simulink model "GuytonModel1986All_R2015a"  (R2015a)
settings: Solver=ode15s  StartTime=0  StopTime=383040  FixedStep=0.03  MaxStep=360  RelTol=1e-3
libraries: simulink x3
(part 4 of 5)

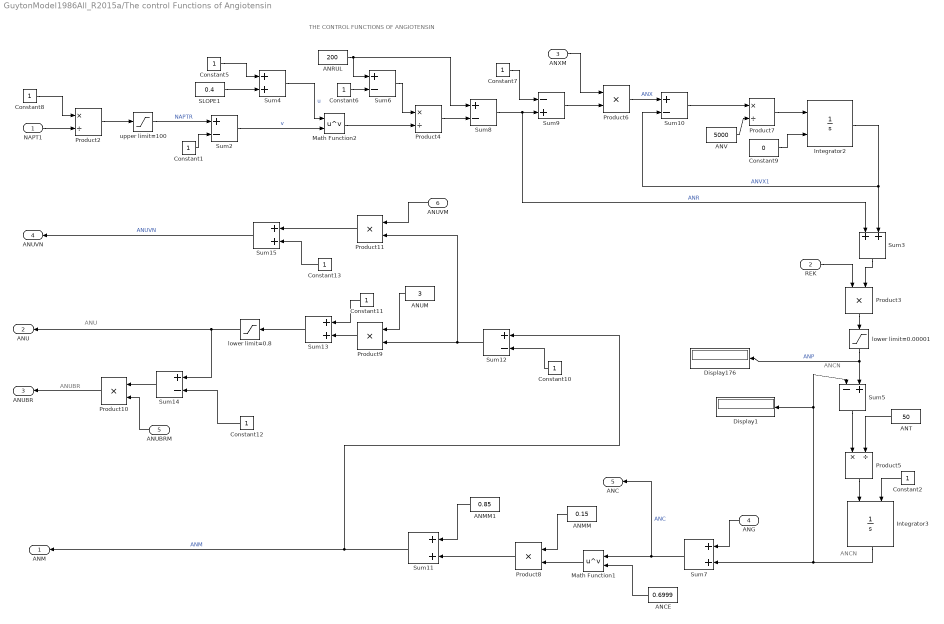
== system GuytonModel1986All_R2015a/The control Functions of Angiotensin ==
  note: THE CONTROL FUNCTIONS OF ANGIOTENSIN
  note: ANCN
  note: ANCN
  note: ANUBR
  note: ANU
  NAPT1 : Inport
  REK : Inport  Port=2
  ANXM : Inport  Port=3
  ANG : Inport  Port=4
  ANUBRM : Inport  Port=5
  ANUVM : Inport  Port=6
  ANCE : Constant  Value=0.6999
  ANMM : Constant  Value=0.15
  ANMM1 : Constant  Value=0.85
  ANRUL : Constant  Value=200
  ANT : Constant  Value=50
  ANUM : Constant  Value=3
  ANV : Constant  Value=5000
  Constant{1..2,5..8,10..13} (10 alike) : Constant
  Constant9 : Constant  Value=0
  Display1 : Display
  Display176 : Display
  Integrator2 : Integrator  InitialConditionSource=external
  Integrator3 : Integrator  InitialConditionSource=external
  Math Function1 : Math  Operator=pow  SaturateOnIntegerOverflow=on
  Math Function2 : Math  Operator=pow  SaturateOnIntegerOverflow=on
  Product{3,6,8..11} (6 alike) : Product  SaturateOnIntegerOverflow=on  RndMeth=Zero  InputSameDT=on  OutDataTypeStr=Inherit: Same as first input
  Product{2,4..5,7} (4 alike) : Product  Inputs=*/  SaturateOnIntegerOverflow=on  RndMeth=Zero  InputSameDT=on  OutDataTypeStr=Inherit: Same as first input
  SLOPE1 : Constant  Value=0.4
  Sum{2,6,8,10,12,14} (6 alike) : Sum  Inputs=+-  SaturateOnIntegerOverflow=on  InputSameDT=on  OutDataTypeStr=Inherit: Same as first input
  Sum11 : Sum  SaturateOnIntegerOverflow=on  InputSameDT=on  OutDataTypeStr=Inherit: Same as first input
  Sum13 : Sum  Inputs=2  SaturateOnIntegerOverflow=on  InputSameDT=on  OutDataTypeStr=Inherit: Same as first input
  Sum15 : Sum  SaturateOnIntegerOverflow=on  InputSameDT=on  OutDataTypeStr=Inherit: Same as first input
  Sum3 : Sum  Inputs=2  SaturateOnIntegerOverflow=on  InputSameDT=on  OutDataTypeStr=Inherit: Same as first input
  Sum4 : Sum  Inputs=2  SaturateOnIntegerOverflow=on  InputSameDT=on  OutDataTypeStr=Inherit: Same as first input
  Sum5 : Sum  Inputs=-+  SaturateOnIntegerOverflow=on  InputSameDT=on  OutDataTypeStr=Inherit: Same as first input
  Sum7 : Sum  SaturateOnIntegerOverflow=on  InputSameDT=on  OutDataTypeStr=Inherit: Same as first input
  Sum9 : Sum  Inputs=-+  SaturateOnIntegerOverflow=on  InputSameDT=on  OutDataTypeStr=Inherit: Same as first input
  lower limit=0.00001 : Saturate  UpperLimit=inf  LowerLimit=0.00001  LinearizeAsGain=off
  lower limit=0.8 : Saturate  UpperLimit=inf  LowerLimit=0.8  LinearizeAsGain=off
  "upper limit=100 " : Saturate  UpperLimit=100  LowerLimit=-inf  LinearizeAsGain=off
  ANM : Outport
  ANU : Outport  Port=2
  ANUBR : Outport  Port=3
  ANUVN : Outport  Port=4
  ANC : Outport  Port=5
  wires:
  NAPT1/1 -> Product2/2
  Constant8/1 -> Product2/1
  Product2/1 -> "upper limit=100 "/1
  "upper limit=100 "/1 -> Sum2/1  "NAPTR"
  Constant1/1 -> Sum2/2
  SLOPE1/1 -> Sum4/2
  Constant5/1 -> Sum4/1
  Sum4/1 -> Math Function2/1  "u"
  Sum2/1 -> Math Function2/2  "v"
  Constant6/1 -> Sum6/2
  ANRUL/1 -> Sum6/1, Sum8/1
  Math Function2/1 -> Product4/2
  Sum6/1 -> Product4/1
  Product4/1 -> Sum8/2
  Sum8/1 -> Sum9/2, Sum3/1  "ANR"
  Constant7/1 -> Sum9/1
  Sum9/1 -> Product6/2
  ANXM/1 -> Product6/1
  Product6/1 -> Sum10/1  "ANX"
  Sum10/1 -> Product7/1
  ANV/1 -> Product7/2
  Product7/1 -> Integrator2/1
  Constant9/1 -> Integrator2/2
  Integrator2/1 -> Sum10/2, Sum3/2  "ANVX1"
  Sum3/1 -> Product3/2
  REK/1 -> Product3/1
  Product3/1 -> lower limit=0.00001/1
  lower limit=0.00001/1 -> Sum5/2, Display176/1  "ANP"
  Sum5/1 -> Product5/1
  ANT/1 -> Product5/2
  Constant2/1 -> Integrator3/2
  Product5/1 -> Integrator3/1
  Integrator3/1 -> Sum7/2, Sum5/1, Display1/1
  ANG/1 -> Sum7/1
  Sum7/1 -> Math Function1/1, ANC/1  "ANC"
  ANCE/1 -> Math Function1/2
  Math Function1/1 -> Product8/2
  ANMM/1 -> Product8/1
  Product8/1 -> Sum11/2
  ANMM1/1 -> Sum11/1
  Sum11/1 -> Sum12/1, ANM/1  "ANM"
  Constant10/1 -> Sum12/2
  Sum12/1 -> Product9/2, Product11/2
  ANUM/1 -> Product9/1
  Product9/1 -> Sum13/2
  Constant11/1 -> Sum13/1
  Sum13/1 -> lower limit=0.8/1
  lower limit=0.8/1 -> Sum14/1, ANU/1
  Constant12/1 -> Sum14/2
  Sum14/1 -> Product10/1
  ANUBRM/1 -> Product10/2
  Product10/1 -> ANUBR/1
  ANUVM/1 -> Product11/1
  Constant13/1 -> Sum15/2
  Product11/1 -> Sum15/1
  Sum15/1 -> ANUVN/1  "ANUVN"

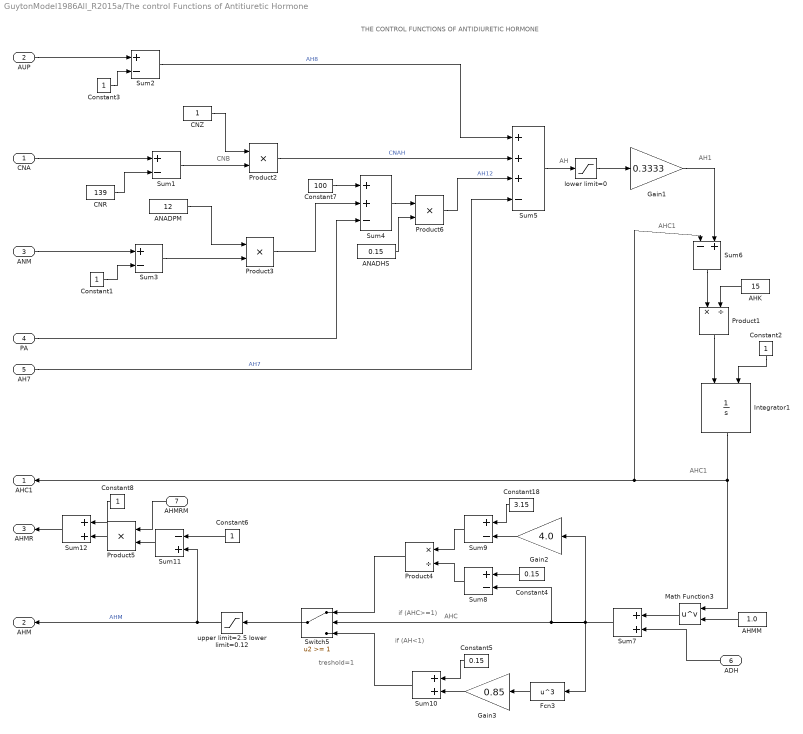
== system GuytonModel1986All_R2015a/The control Functions of Antitiuretic Hormone ==
  note: THE CONTROL FUNCTIONS OF ANTIDIURETIC HORMONE
  note: CNB
  note: AH
  note: AHC1
  note: AHC1
  note: treshold=1
  note: AHC
  note: if (AHC>=1)
  note: if (AH<1)
  note: AH1
  CNA : Inport
  AUP : Inport  Port=2
  ANM : Inport  Port=3
  PA : Inport  Port=4
  AH7 : Inport  Port=5
  ADH : Inport  Port=6
  AHMRM : Inport  Port=7
  AHK : Constant  Value=15
  AHMM : Constant  Value=1.0
  ANADHS : Constant  Value=0.15
  ANADPM : Constant  Value=12
  CNR : Constant  Value=139
  CNZ : Constant
  Constant{1..3,6,8} (5 alike) : Constant
  Constant18 : Constant  Value=3.15
  Constant4 : Constant  Value=0.15
  Constant5 : Constant  Value=0.15
  Constant7 : Constant  Value=100
  Fcn3 : Fcn  Expr=u^3
  Gain1 : Gain  Gain=0.3333  SaturateOnIntegerOverflow=on  OutDataTypeStr=Inherit: Same as input  ParamDataTypeStr=Inherit: Same as input
  Gain2 : Gain  Gain=4.0  SaturateOnIntegerOverflow=on  OutDataTypeStr=Inherit: Same as input  ParamDataTypeStr=Inherit: Same as input
  Gain3 : Gain  Gain=0.85  SaturateOnIntegerOverflow=on  OutDataTypeStr=Inherit: Same as input  ParamDataTypeStr=Inherit: Same as input
  Integrator1 : Integrator  InitialConditionSource=external
  Math Function3 : Math  Operator=pow  SaturateOnIntegerOverflow=on
  Product1 : Product  Inputs=*/  SaturateOnIntegerOverflow=on  RndMeth=Zero  InputSameDT=on  OutDataTypeStr=Inherit: Same as first input
  Product{2..3,5..6} (4 alike) : Product  SaturateOnIntegerOverflow=on  RndMeth=Zero  InputSameDT=on  OutDataTypeStr=Inherit: Same as first input
  Product4 : Product  Inputs=*/  SaturateOnIntegerOverflow=on  RndMeth=Zero  InputSameDT=on  OutDataTypeStr=Inherit: Same as first input
  Sum{1..3,8..9} (5 alike) : Sum  Inputs=+-  SaturateOnIntegerOverflow=on  InputSameDT=on  OutDataTypeStr=Inherit: Same as first input
  Sum10 : Sum  Inputs=2  SaturateOnIntegerOverflow=on  InputSameDT=on  OutDataTypeStr=Inherit: Same as first input
  Sum11 : Sum  Inputs=-+  SaturateOnIntegerOverflow=on  InputSameDT=on  OutDataTypeStr=Inherit: Same as first input
  Sum12 : Sum  Inputs=2  SaturateOnIntegerOverflow=on  InputSameDT=on  OutDataTypeStr=Inherit: Same as first input
  Sum4 : Sum  Inputs=++-  SaturateOnIntegerOverflow=on  InputSameDT=on  OutDataTypeStr=Inherit: Same as first input
  Sum5 : Sum  Inputs=+++-  SaturateOnIntegerOverflow=on  InputSameDT=on  OutDataTypeStr=Inherit: Same as first input
  Sum6 : Sum  Inputs=-+  SaturateOnIntegerOverflow=on  InputSameDT=on  OutDataTypeStr=Inherit: Same as first input
  Sum7 : Sum  Inputs=2  SaturateOnIntegerOverflow=on  InputSameDT=on  OutDataTypeStr=Inherit: Same as first input
  Switch5 : Switch  Threshold=1  SaturateOnIntegerOverflow=on  InputSameDT=on
  "lower limit=0 " : Saturate  UpperLimit=inf  LowerLimit=0  LinearizeAsGain=off
  "upper limit=2.5 lower limit=0.12 " : Saturate  UpperLimit=inf  LowerLimit=0  LinearizeAsGain=off
  AHC1 : Outport
  AHM : Outport  Port=2
  AHMR : Outport  Port=3
  wires:
  CNR/1 -> Sum1/2
  CNA/1 -> Sum1/1
  Sum1/1 -> Product2/2
  CNZ/1 -> Product2/1
  Constant3/1 -> Sum2/2
  AUP/1 -> Sum2/1
  Constant1/1 -> Sum3/2
  ANM/1 -> Sum3/1
  Sum3/1 -> Product3/2
  ANADPM/1 -> Product3/1
  Product3/1 -> Sum4/2
  PA/1 -> Sum4/3
  Sum2/1 -> Sum5/1  "AH8"
  Constant7/1 -> Sum4/1
  Product2/1 -> Sum5/2  "CNAH"
  AH7/1 -> Sum5/4  "AH7"
  Sum5/1 -> "lower limit=0 "/1
  "lower limit=0 "/1 -> Gain1/1
  Constant2/1 -> Integrator1/2
  AHK/1 -> Product1/2
  Sum6/1 -> Product1/1
  Product1/1 -> Integrator1/1
  Integrator1/1 -> Sum6/1, AHC1/1, Math Function3/1
  Gain1/1 -> Sum6/2
  AHMM/1 -> Math Function3/2
  Math Function3/1 -> Sum7/1
  ADH/1 -> Sum7/2
  Sum7/1 -> Switch5/2, Sum8/2, Gain2/1, Fcn3/1
  Constant4/1 -> Sum8/1
  Gain2/1 -> Sum9/2
  Constant18/1 -> Sum9/1
  Sum9/1 -> Product4/1
  Sum8/1 -> Product4/2
  Product4/1 -> Switch5/1
  Fcn3/1 -> Gain3/1
  Gain3/1 -> Sum10/2
  Constant5/1 -> Sum10/1
  Sum10/1 -> Switch5/3
  Switch5/1 -> "upper limit=2.5 lower limit=0.12 "/1
  "upper limit=2.5 lower limit=0.12 "/1 -> AHM/1, Sum11/2  "AHM"
  Constant6/1 -> Sum11/1
  Sum11/1 -> Product5/2
  AHMRM/1 -> Product5/1
  Product5/1 -> Sum12/2
  Constant8/1 -> Sum12/1
  Sum12/1 -> AHMR/1
  Sum4/1 -> Product6/1
  Product6/1 -> Sum5/3  "AH12"
  ANADHS/1 -> Product6/2

== system GuytonModel1986All_R2015a/The volume receptor feedback mechanism ==
  note: PRA
  note: AHZ1
  note: ATRVFB
  note: ATRRFB
  note: AH7
  note: Dumping
  note: The volume receptor feedback mechanism
  PRA : Inport
  ATRVFBM : Inport  Port=2
  ATRRFBM : Inport  Port=3
  "AH10 " : Constant  Value=0.333
  AH11 : Constant  Value=1000
  AH9 : Constant
  AHY : Integrator  InitialConditionSource=external
  AHY0 : Constant  Value=0
  AHY1 : Constant  Value=0.1
  AHZ1=(Abs(PRA))^AH10 : Math  Operator=pow  SaturateOnIntegerOverflow=on
  "ATRVFB " : Integrator  InitialConditionSource=external
  ATRVFB0 : Constant  Value=0
  ATRVFB1 : Constant  Value=0.1
  Abs : Abs  SaturateOnIntegerOverflow=on
  Constant12 : Constant
  Gain1 : Gain  Gain=-1  SaturateOnIntegerOverflow=on  OutDataTypeStr=Inherit: Same as input  ParamDataTypeStr=Inherit: Same as input
  Product{1,4..6} (4 alike) : Product  SaturateOnIntegerOverflow=on  RndMeth=Zero  InputSameDT=on  OutDataTypeStr=Inherit: Same as first input
  Product9 : Product  Inputs=*/  SaturateOnIntegerOverflow=on  RndMeth=Zero  InputSameDT=on  OutDataTypeStr=Inherit: Same as first input
  Sum1 : Sum  Inputs=+-  SaturateOnIntegerOverflow=on  InputSameDT=on  OutDataTypeStr=Inherit: Same as first input
  Sum6 : Sum  Inputs=+-  SaturateOnIntegerOverflow=on  InputSameDT=on  OutDataTypeStr=Inherit: Same as first input
  Sum7 : Sum  SaturateOnIntegerOverflow=on  InputSameDT=on  OutDataTypeStr=Inherit: Same as first input
  Sum9 : Sum  Inputs=+-  SaturateOnIntegerOverflow=on  InputSameDT=on  OutDataTypeStr=Inherit: Same as first input
  if (ATRRFB)>=0.!) ATRRFB=ATRRFB else ATRRFB= 0.1 : Switch  Threshold=0.1  SaturateOnIntegerOverflow=on  InputSameDT=on
  "if (PRA>=0) AHZ2=AHZ1 else AHZ2= -AHZ1  " : Switch  SaturateOnIntegerOverflow=on  InputSameDT=on
  AH7 : Outport
  ATRVFB : Outport  Port=2
  ATRRFB : Outport  Port=3
  wires:
  Product1/1 -> "ATRVFB "/1
  ATRVFB1/1 -> Product1/2
  "ATRVFB "/1 -> Sum1/2, ATRVFB/1
  Sum1/1 -> Product1/1
  ATRVFB0/1 -> "ATRVFB "/2
  "AH10 "/1 -> AHZ1=(Abs(PRA))^AH10/2
  Abs/1 -> AHZ1=(Abs(PRA))^AH10/1
  AH11/1 -> Product9/2
  AHY0/1 -> AHY/2
  ATRRFBM/1 -> Product5/1
  PRA/1 -> "if (PRA>=0) AHZ2=AHZ1 else AHZ2= -AHZ1  "/2, Abs/1  "PRA"
  Product6/1 -> Sum1/1
  ATRVFBM/1 -> Product6/1
  Constant12/1 -> Sum7/1
  Product5/1 -> Sum7/2
  AH9/1 -> Product4/1
  Gain1/1 -> "if (PRA>=0) AHZ2=AHZ1 else AHZ2= -AHZ1  "/3  "-AHZ1"
  AHZ1=(Abs(PRA))^AH10/1 -> "if (PRA>=0) AHZ2=AHZ1 else AHZ2= -AHZ1  "/1, Gain1/1  "AHZ1"
  Sum6/1 -> AH7/1, Product6/2, Product5/2
  Product4/1 -> Sum9/1, Sum6/1  "AHZ"
  Sum9/1 -> Product9/1
  "if (PRA>=0) AHZ2=AHZ1 else AHZ2= -AHZ1  "/1 -> Product4/2
  AHY/1 -> Sum9/2, Sum6/2
  Product9/1 -> AHY/1
  AHY1/1 -> if (ATRRFB)>=0.!) ATRRFB=ATRRFB else ATRRFB= 0.1/3
  Sum7/1 -> if (ATRRFB)>=0.!) ATRRFB=ATRRFB else ATRRFB= 0.1/2, if (ATRRFB)>=0.!) ATRRFB=ATRRFB else ATRRFB= 0.1/1
  if (ATRRFB)>=0.!) ATRRFB=ATRRFB else ATRRFB= 0.1/1 -> ATRRFB/1

== system GuytonModel1986All_R2015a/Thirst, Drinking and Salt Appetite ==
  note: If TVD <0 then TVD=DR
  note: If STHENABLED <0 then STH=1
  note: TVZ
  note: ANMTH
  note: THIRST, DRINKING AND SALT APPETITE
  POT : Inport
  AHC1 : Inport  Port=2
  ANM : Inport  Port=3
  DR : Inport  Port=4
  STHENABLED : Inport  Port=5
  TVDENABLED : Inport  Port=6
  AHTHM : Constant  Value=2
  ANMTM : Constant  Value=1.5
  Constant{1..3,8} (4 alike) : Constant
  Constant4 : Constant  Value=0.001
  Display4 : Display
  Gain1 : Gain  Gain=0.001  SaturateOnIntegerOverflow=on  OutDataTypeStr=Inherit: Same as input  ParamDataTypeStr=Inherit: Same as input
  Gain2 : Gain  Gain=0.001  SaturateOnIntegerOverflow=on  OutDataTypeStr=Inherit: Same as input  ParamDataTypeStr=Inherit: Same as input
  Integrator1 : Integrator  InitialConditionSource=external
  Product{1..5} (5 alike) : Product  SaturateOnIntegerOverflow=on  RndMeth=Zero  InputSameDT=on  OutDataTypeStr=Inherit: Same as first input
  Sum1 : Sum  Inputs=+-  SaturateOnIntegerOverflow=on  InputSameDT=on  OutDataTypeStr=Inherit: Same as first input
  Sum2 : Sum  Inputs=+-  SaturateOnIntegerOverflow=on  InputSameDT=on  OutDataTypeStr=Inherit: Same as first input
  Sum3 : Sum  SaturateOnIntegerOverflow=on  InputSameDT=on  OutDataTypeStr=Inherit: Same as first input
  Sum5 : Sum  SaturateOnIntegerOverflow=on  InputSameDT=on  OutDataTypeStr=Inherit: Same as first input
  Sum6 : Sum  Inputs=+-  SaturateOnIntegerOverflow=on  InputSameDT=on  OutDataTypeStr=Inherit: Same as first input
  Sum7 : Sum  Inputs=-++  SaturateOnIntegerOverflow=on  InputSameDT=on  OutDataTypeStr=Inherit: Same as first input
  TRESHOLD=0 : Switch  Criteria=u2 > Threshold
  "TRESHOLD=0 " : Switch  Criteria=u2 > Threshold
  TVDDL : Constant  Value=30
  Z10 : Constant  Value=8.25
  Z11 : Constant  Value=4
  lower limit=0 : Saturate  UpperLimit=inf  LowerLimit=0  LinearizeAsGain=off
  "lower limit=0 " : Saturate  UpperLimit=inf  LowerLimit=0  LinearizeAsGain=off
  "upper limit=8 lower limit=1 " : Saturate  UpperLimit=8  LowerLimit=1  LinearizeAsGain=off
  STH : Outport
  TVD : Outport  Port=2
  wires:
  TVDENABLED/1 -> "TRESHOLD=0 "/2
  "TRESHOLD=0 "/1 -> TVD/1
  STHENABLED/1 -> TRESHOLD=0/2
  Constant3/1 -> TRESHOLD=0/3
  TRESHOLD=0/1 -> STH/1
  Product5/1 -> Integrator1/1
  Sum7/1 -> Product5/1
  Integrator1/1 -> "TRESHOLD=0 "/1, Sum7/1  "TVD"
  DR/1 -> "TRESHOLD=0 "/3, Sum7/3
  TVDDL/1 -> Product5/2
  Constant4/1 -> Integrator1/2
  "lower limit=0 "/1 -> Sum7/2  "TVZ"
  Sum5/1 -> "lower limit=0 "/1
  Gain2/1 -> Sum5/1
  Product4/1 -> Gain2/1
  ANMTM/1 -> Product4/1
  Sum6/1 -> Product4/2
  ANM/1 -> Sum6/1
  Constant2/1 -> Sum6/2
  lower limit=0/1 -> Sum5/2  "ANMTH"
  Product3/1 -> lower limit=0/1  "AHTH"
  Gain1/1 -> Product3/2
  Sum3/1 -> Product3/1
  Constant1/1 -> Sum3/2
  Product2/1 -> Sum3/1
  AHTHM/1 -> Product2/1
  Sum2/1 -> Product2/2
  AHC1/1 -> Sum2/1
  Constant8/1 -> Sum2/2
  "upper limit=8 lower limit=1 "/1 -> TRESHOLD=0/1, Gain1/1
  Product1/1 -> Display4/1, "upper limit=8 lower limit=1 "/1
  Z11/1 -> Product1/1
  Sum1/1 -> Product1/2
  Z10/1 -> Sum1/1
  POT/1 -> Sum1/2

== system GuytonModel1986All_R2015a/Unstressed volume in systemic venous tree ==
  note: Unstressed volume in systemic venous tree
  VVR : Inport
  ANU : Inport  Port=2
  ANY : Inport  Port=3
  VV6 : Inport  Port=4
  VV7 : Inport  Port=5
  ATRVFB : Inport  Port=6
  Add1 : Sum  Inputs=5
  Add21 : Sum  Inputs=|+-
  Divide1 : Product
  PR1LL1 : Constant
  VVS0 : Outport
  wires:
  Add1/1 -> VVS0/1
  VV6/1 -> Add1/3
  VV7/1 -> Add1/4
  ATRVFB/1 -> Add1/5
  VVR/1 -> Add1/1
  Divide1/1 -> Add1/2  "VV_ANU"
  ANY/1 -> Divide1/2
  Add21/1 -> Divide1/1
  PR1LL1/1 -> Add21/2
  ANU/1 -> Add21/1

== system GuytonModel1986All_R2015a/Urea ==
  note: UREA
  URFORM : Inport
  UROD : Inport  Port=2
  VTW : Inport  Port=3
  PLURCNORM : Inport  Port=4
  Integrator2 : Integrator  InitialConditionSource=external
  Product1 : Product  SaturateOnIntegerOverflow=on  RndMeth=Zero  InputSameDT=on  OutDataTypeStr=Inherit: Same as first input
  Product3 : Product  Inputs=*/  SaturateOnIntegerOverflow=on  RndMeth=Zero  InputSameDT=on  OutDataTypeStr=Inherit: Same as first input
  Sum1 : Sum  Inputs=+-  SaturateOnIntegerOverflow=on  InputSameDT=on  OutDataTypeStr=Inherit: Same as first input
  PLURC : Outport
  PLUR : Outport  Port=2
  wires:
  Product3/1 -> PLURC/1
  Integrator2/1 -> PLUR/1, Product3/1  "PLUR"
  Sum1/1 -> Integrator2/1
  UROD/1 -> Sum1/2  "UROD"
  URFORM/1 -> Sum1/1  "URFORM"
  Product1/1 -> Integrator2/2
  PLURCNORM/1 -> Product1/1
  VTW/1 -> Product3/2, Product1/2  "VTW"

== system GuytonModel1986All_R2015a/Urea and Water Excretion ==
  note: WATER AND UREA EXCRETION
  note: OSMOPN0
  PLURC : Inport
  GFN : Inport  Port=2
  NODN : Inport  Port=3
  KODN : Inport  Port=4
  AHM : Inport  Port=5
  REK : Inport  Port=6
  Constant1 : Constant  Value=2
  Constant2 : Constant  Value=0.56
  Constant3 : Constant  Value=560
  Constant4 : Constant  Value=3.84
  Constant5 : Constant  Value=360
  Product1 : Product  SaturateOnIntegerOverflow=on  RndMeth=Zero  InputSameDT=on  OutDataTypeStr=Inherit: Same as first input
  Product11 : Product  Inputs=4  SaturateOnIntegerOverflow=on  RndMeth=Zero  InputSameDT=on  OutDataTypeStr=Inherit: Same as first input
  Product2 : Product  Inputs=//*  SaturateOnIntegerOverflow=on  RndMeth=Zero  InputSameDT=on  OutDataTypeStr=Inherit: Same as first input
  Product3 : Product  Inputs=*/  SaturateOnIntegerOverflow=on  RndMeth=Zero  InputSameDT=on  OutDataTypeStr=Inherit: Same as first input
  Product4 : Product  SaturateOnIntegerOverflow=on  RndMeth=Zero  InputSameDT=on  OutDataTypeStr=Inherit: Same as first input
  Product5 : Product  SaturateOnIntegerOverflow=on  RndMeth=Zero  InputSameDT=on  OutDataTypeStr=Inherit: Same as first input
  Sum1 : Sum  SaturateOnIntegerOverflow=on  InputSameDT=on  OutDataTypeStr=Inherit: Same as first input
  Sum2 : Sum  Inputs=+-  SaturateOnIntegerOverflow=on  InputSameDT=on  OutDataTypeStr=Inherit: Same as first input
  Sum3 : Sum  SaturateOnIntegerOverflow=on  InputSameDT=on  OutDataTypeStr=Inherit: Same as first input
  Sum4 : Sum  SaturateOnIntegerOverflow=on  InputSameDT=on  OutDataTypeStr=Inherit: Same as first input
  lower limit 0.0 : Saturate  UpperLimit=inf  LowerLimit=0  LinearizeAsGain=off
  upper limit 0.56 : Saturate  UpperLimit=0.56  LowerLimit=-inf  LinearizeAsGain=off
  UROD : Outport
  VUDN : Outport  Port=2
  VUD : Outport  Port=3
  wires:
  Constant4/1 -> Product11/4
  GFN/1 -> Product11/3, Product11/2
  PLURC/1 -> Product11/1  "PLURC"
  NODN/1 -> Sum4/1
  KODN/1 -> Sum4/2
  Sum4/1 -> Product1/2
  Constant1/1 -> Product1/1
  Product1/1 -> Sum1/2
  Product11/1 -> Product4/2, Sum1/1  "DTURI"
  Sum1/1 -> Sum2/1, upper limit 0.56/1  "OSMOPN"
  Constant2/1 -> Sum2/2
  Sum2/1 -> lower limit 0.0/1  "OSMOP1"
  upper limit 0.56/1 -> Product2/3
  lower limit 0.0/1 -> Product3/1  "OSMOP1"
  AHM/1 -> Product2/2
  Constant3/1 -> Product2/1
  Product2/1 -> Sum3/1  "VUD0"
  Constant5/1 -> Product3/2
  Product3/1 -> Sum3/2  "VUDN1"
  Sum3/1 -> VUDN/1, Product5/2
  Product4/1 -> UROD/1
  REK/1 -> Product4/1, Product5/1
  Product5/1 -> VUD/1

== system GuytonModel1986All_R2015a/Autonomic Contorl of the Circulation/AUB calculation ==
  note: when PA1<40:            AUB=1.85718
      | when  40>PA1<170:  AUB=0.01426*(170-PA1)
      | when PA1>=170:        AUB=0
  note: AUB calculation
  PA1 : Inport
  Constant1 : Constant  Value=170
  Constant2 : Constant  Value=0
  Constant3 : Constant  Value=1.85718
  Gain1 : Gain  Gain=0.014286  SaturateOnIntegerOverflow=on  OutDataTypeStr=Inherit: Same as input  ParamDataTypeStr=Inherit: Same as input
  Sum1 : Sum  Inputs=+-  SaturateOnIntegerOverflow=on  InputSameDT=on  OutDataTypeStr=Inherit: Same as first input
  if (PA1>=170) AUB1=0 else AUB1=0.014286*(80-PA1) : Switch  Threshold=170  SaturateOnIntegerOverflow=on  InputSameDT=on
  "if (PA1>=40) {AUB=AUB1) else AUB=1.859" : Switch  Threshold=40  SaturateOnIntegerOverflow=on  InputSameDT=on
  AUB : Outport  InitialOutput=0
  wires:
  "if (PA1>=40) {AUB=AUB1) else AUB=1.859"/1 -> AUB/1
  Constant3/1 -> "if (PA1>=40) {AUB=AUB1) else AUB=1.859"/3
  if (PA1>=170) AUB1=0 else AUB1=0.014286*(80-PA1)/1 -> "if (PA1>=40) {AUB=AUB1) else AUB=1.859"/1  "AUB1"
  Constant2/1 -> if (PA1>=170) AUB1=0 else AUB1=0.014286*(80-PA1)/1
  Gain1/1 -> if (PA1>=170) AUB1=0 else AUB1=0.014286*(80-PA1)/3
  PA1/1 -> "if (PA1>=40) {AUB=AUB1) else AUB=1.859"/2, if (PA1>=170) AUB1=0 else AUB1=0.014286*(80-PA1)/2, Sum1/2  "PA1"
  Sum1/1 -> Gain1/1
  Constant1/1 -> Sum1/1

== system GuytonModel1986All_R2015a/Autonomic Contorl of the Circulation/AUC calculation ==
  note: when PA1<40:          AUCC=1.2
      | when  40>PA1<80:  AUC=0.03*(80-PA1)
      | when PA1>=80:        AUC=0
  note: AUC calculation
  PA1 : Inport
  Constant1 : Constant  Value=80
  Constant2 : Constant  Value=0
  Constant3 : Constant  Value=1.2
  Gain1 : Gain  Gain=0.03  SaturateOnIntegerOverflow=on  OutDataTypeStr=Inherit: Same as input  ParamDataTypeStr=Inherit: Same as input
  Sum1 : Sum  Inputs=+-  SaturateOnIntegerOverflow=on  InputSameDT=on  OutDataTypeStr=Inherit: Same as first input
  "if (PA1>=40) {AUC=AUC1) else AUC=1.2" : Switch  Threshold=40  SaturateOnIntegerOverflow=on  InputSameDT=on
  if (PA1>=80) AUC1=0 else AUC1=0.03*(80-PA1) : Switch  Threshold=80  SaturateOnIntegerOverflow=on  InputSameDT=on
  AUC : Outport  InitialOutput=0
  wires:
  Constant1/1 -> Sum1/1
  Sum1/1 -> Gain1/1
  PA1/1 -> Sum1/2, if (PA1>=80) AUC1=0 else AUC1=0.03*(80-PA1)/2, "if (PA1>=40) {AUC=AUC1) else AUC=1.2"/2  "PA1"
  Gain1/1 -> if (PA1>=80) AUC1=0 else AUC1=0.03*(80-PA1)/3
  Constant2/1 -> if (PA1>=80) AUC1=0 else AUC1=0.03*(80-PA1)/1
  if (PA1>=80) AUC1=0 else AUC1=0.03*(80-PA1)/1 -> "if (PA1>=40) {AUC=AUC1) else AUC=1.2"/1  "AUC1"
  Constant3/1 -> "if (PA1>=40) {AUC=AUC1) else AUC=1.2"/3
  "if (PA1>=40) {AUC=AUC1) else AUC=1.2"/1 -> AUC/1

== system GuytonModel1986All_R2015a/Autonomic Contorl of the Circulation/AUN calculation ==
  note: when PA1<20:           AUN=6
      | when  20>PA1<50:  AUN=0.2*(50-PA1)
      | when PA1>=50:        AUN=0
  note: AUN calculation
  PA1 : Inport
  Constant1 : Constant  Value=50
  Constant2 : Constant  Value=0
  Constant3 : Constant  Value=6
  Gain1 : Gain  Gain=0.2  SaturateOnIntegerOverflow=on  OutDataTypeStr=Inherit: Same as input  ParamDataTypeStr=Inherit: Same as input
  Sum1 : Sum  Inputs=+-  SaturateOnIntegerOverflow=on  InputSameDT=on  OutDataTypeStr=Inherit: Same as first input
  "if (PA1>=20) {AUN=AUN1) else AUN=6" : Switch  Threshold=20  SaturateOnIntegerOverflow=on  InputSameDT=on
  if (PA1>=50) AUB1=0 else AUN1=0.2*(50-PA1) : Switch  Threshold=50  SaturateOnIntegerOverflow=on  InputSameDT=on
  AUN : Outport  InitialOutput=0
  wires:
  Constant1/1 -> Sum1/1
  Sum1/1 -> Gain1/1
  PA1/1 -> Sum1/2, if (PA1>=50) AUB1=0 else AUN1=0.2*(50-PA1)/2, "if (PA1>=20) {AUN=AUN1) else AUN=6"/2  "PA1"
  Gain1/1 -> if (PA1>=50) AUB1=0 else AUN1=0.2*(50-PA1)/3
  Constant2/1 -> if (PA1>=50) AUB1=0 else AUN1=0.2*(50-PA1)/1
  if (PA1>=50) AUB1=0 else AUN1=0.2*(50-PA1)/1 -> "if (PA1>=20) {AUN=AUN1) else AUN=6"/1  "AUN1"
  Constant3/1 -> "if (PA1>=20) {AUN=AUN1) else AUN=6"/3
  "if (PA1>=20) {AUN=AUN1) else AUN=6"/1 -> AUN/1

== system GuytonModel1986All_R2015a/Myogenic Autoregulation/function MyogenResp(PDIFF) - spline interpolation ==
  x : Inport
  xySlope : Inport  Port=2
  Constant : Constant  Value=-10
  If : If  IfExpression=u1 >=0  ShowElse=off
  If Action Subsystem : Subsystem  TreatAsAtomicUnit=on
  Memory init =0 : Memory
  Subsystem : Subsystem
  y : Outport
  wires:
  Memory init =0/1 -> If/1
  Constant/1 -> Memory init =0/1
  If/1 -> If Action Subsystem/Action  "init=0"
  x/1 -> Subsystem/1(x)
  xySlope/1 -> If Action Subsystem/1(X1)
  Subsystem/1(y) -> y/1
  If Action Subsystem/1(aa) -> Subsystem/2(aa)

== system GuytonModel1986All_R2015a/Myogenic Autoregulation of Afferent Arteriole/function MyogenResp(PDIFF) - spline interpolation ==
  x : Inport
  xySlope : Inport  Port=2
  Constant : Constant  Value=-10
  If : If  IfExpression=u1 >=0  ShowElse=off
  If Action Subsystem : Subsystem  TreatAsAtomicUnit=on
  Memory init =0 : Memory
  Subsystem : Subsystem
  y : Outport
  wires:
  Memory init =0/1 -> If/1
  Constant/1 -> Memory init =0/1
  If/1 -> If Action Subsystem/Action  "init=0"
  x/1 -> Subsystem/1(x)
  xySlope/1 -> If Action Subsystem/1(X1)
  Subsystem/1(y) -> y/1
  If Action Subsystem/1(aa) -> Subsystem/2(aa)

== system GuytonModel1986All_R2015a/Myogenic Autoregulation/function MyogenResp(PDIFF) - spline interpolation/If Action Subsystem ==
  X1 : Inport
  Action Port : ActionPort  ActionType=then
  Cubica : Subsystem
      mask help: Cubica
      mask Help: Calculates vector of coeffitients of cubica spline from points of coordinate and slope of experimental curve
      mask Display: disp('C U B I C A\n\nINPUTS :\nx1, y1   -  first point of coordinate\nSlope1 - slope (dy/dx) at point x1,y1 \n x2, y2   -  second point of coordinate\nSlope2 - slope (dy/dx) at point x2,y2 \n\nOUTPUTS :\na1, a2, a3, a4 - vector of coeffitients\n a1, a2, a3, a4 of cubica:\n  y = a1*x^3 + a2*x^2 + a3*x + a4')
  Cubica1 : Subsystem
      mask help: Cubica
      mask Help: Calculates vector of coeffitients of cubica spline from points of coordinate and slope of experimental curve
      mask Display: disp('C U B I C A\n\nINPUTS :\nx1, y1   -  first point of coordinate\nSlope1 - slope (dy/dx) at point x1,y1 \n x2, y2   -  second point of coordinate\nSlope2 - slope (dy/dx) at point x2,y2 \n\nOUTPUTS :\na1, a2, a3, a4 - vector of coeffitients\n a1, a2, a3, a4 of cubica:\n  y = a1*x^3 + a2*x^2 + a3*x + a4')
  Demux : Demux  Outputs=9
  Mux : Mux  Inputs=15
  Product : Product  SaturateOnIntegerOverflow=on  InputSameDT=on  OutDataTypeStr=Inherit: Same as first input
  Product1 : Product  SaturateOnIntegerOverflow=on  InputSameDT=on  OutDataTypeStr=Inherit: Same as first input
  Sum : Sum  Inputs=+-  SaturateOnIntegerOverflow=on  InputSameDT=on  OutDataTypeStr=Inherit: Same as first input
  Sum2 : Sum  Inputs=+-  SaturateOnIntegerOverflow=on  InputSameDT=on  OutDataTypeStr=Inherit: Same as first input
  aa : Outport
  wires:
  Demux/1 -> Product/1, Cubica/1(X1), Mux/1  "xySlope1"
  Demux/7 -> Product1/1, Cubica1/4(X2), Mux/3  "xySlope7"
  Demux/3 -> Product/2, Mux/4, Cubica/3(Slope1)  "xySlope3"
  Demux/2 -> Sum/1, Cubica/2(Y1)  "xySlope2"
  Demux/5 -> Cubica/5(Y2), Cubica1/2(Y1)  "xySlope5"
  Demux/6 -> Cubica/6(Slope2), Cubica1/3(Slope1)  "xySlope6"
  Demux/8 -> Sum2/1, Cubica1/5(Y2)  "xySlope8"
  Demux/9 -> Product1/2, Mux/14, Cubica1/6(Slope2)  "xySlope9"
  Demux/4 -> Cubica/4(X2), Cubica1/1(X1), Mux/2  "xySlope4"
  Product/1 -> Sum/2  ";"
  Sum/1 -> Mux/5  "aa)=xyslope(2)-xyslope(3)*xyslope(1)"
  Cubica/1(a1) -> Mux/6
  Cubica/2(a2) -> Mux/7
  Cubica/3(a3) -> Mux/8
  Cubica/4(a4) -> Mux/9
  Cubica1/1(a1) -> Mux/10
  Cubica1/2(a2) -> Mux/11
  Cubica1/3(a3) -> Mux/12
  Cubica1/4(a4) -> Mux/13
  Product1/1 -> Sum2/2
  Sum2/1 -> Mux/15  "aa15=xyslope8-xyslope9*xyslope7"
  X1/1 -> Demux/1
  Mux/1 -> aa/1

== system GuytonModel1986All_R2015a/Myogenic Autoregulation/function MyogenResp(PDIFF) - spline interpolation/Subsystem ==
  x : Inport
  aa : Inport  Port=2
  Demux : Demux  Outputs=15
  If : If  NumInputs=4  IfExpression=u1 <=u2  ElseIfExpressions=u1<=u3,u1<=u4
  If Action Subsystem : Subsystem  TreatAsAtomicUnit=on
  If Action Subsystem1 : Subsystem  TreatAsAtomicUnit=on
  If Action Subsystem2 : Subsystem  TreatAsAtomicUnit=on
  If Action Subsystem3 : Subsystem  TreatAsAtomicUnit=on
  Merge : Merge  Inputs=4
  y : Outport
  wires:
  x/1 -> If Action Subsystem3/1(x), If Action Subsystem2/1(x), If Action Subsystem1/1(x), If Action Subsystem/1(x), If/1
  Demux/1 -> If/2
  Merge/1 -> y/1
  If/1 -> If Action Subsystem/Action
  If/2 -> If Action Subsystem1/Action
  If/3 -> If Action Subsystem2/Action
  Demux/6 -> If Action Subsystem1/2(aa6)
  Demux/7 -> If Action Subsystem1/3(aa7)
  Demux/8 -> If Action Subsystem1/4(aa8)
  Demux/9 -> If Action Subsystem1/5(aa9)
  Demux/10 -> If Action Subsystem2/2(aa10)
  Demux/11 -> If Action Subsystem2/3(aa11)
  Demux/12 -> If Action Subsystem2/4(aa12)
  Demux/13 -> If Action Subsystem2/5(aa13)
  If/4 -> If Action Subsystem3/Action
  Demux/15 -> If Action Subsystem3/3(aa15)
  Demux/14 -> If Action Subsystem3/2(aa14)
  If Action Subsystem3/1(Out1) -> Merge/4
  If Action Subsystem2/1(y) -> Merge/3
  If Action Subsystem1/1(y) -> Merge/2
  If Action Subsystem/1(y) -> Merge/1
  Demux/2 -> If/3
  Demux/3 -> If/4
  Demux/4 -> If Action Subsystem/2(aa4)
  Demux/5 -> If Action Subsystem/3("aa6 ")
  aa/1 -> Demux/1

== system GuytonModel1986All_R2015a/Myogenic Autoregulation of Afferent Arteriole/function MyogenResp(PDIFF) - spline interpolation/If Action Subsystem ==
  X1 : Inport
  Action Port : ActionPort  ActionType=then
  Cubica : Subsystem
      mask help: Cubica
      mask Help: Calculates vector of coeffitients of cubica spline from points of coordinate and slope of experimental curve
      mask Display: disp('C U B I C A\n\nINPUTS :\nx1, y1   -  first point of coordinate\nSlope1 - slope (dy/dx) at point x1,y1 \n x2, y2   -  second point of coordinate\nSlope2 - slope (dy/dx) at point x2,y2 \n\nOUTPUTS :\na1, a2, a3, a4 - vector of coeffitients\n a1, a2, a3, a4 of cubica:\n  y = a1*x^3 + a2*x^2 + a3*x + a4')
  Cubica1 : Subsystem
      mask help: Cubica
      mask Help: Calculates vector of coeffitients of cubica spline from points of coordinate and slope of experimental curve
      mask Display: disp('C U B I C A\n\nINPUTS :\nx1, y1   -  first point of coordinate\nSlope1 - slope (dy/dx) at point x1,y1 \n x2, y2   -  second point of coordinate\nSlope2 - slope (dy/dx) at point x2,y2 \n\nOUTPUTS :\na1, a2, a3, a4 - vector of coeffitients\n a1, a2, a3, a4 of cubica:\n  y = a1*x^3 + a2*x^2 + a3*x + a4')
  Demux : Demux  Outputs=9
  Mux : Mux  Inputs=15
  Product : Product  SaturateOnIntegerOverflow=on  InputSameDT=on  OutDataTypeStr=Inherit: Same as first input
  Product1 : Product  SaturateOnIntegerOverflow=on  InputSameDT=on  OutDataTypeStr=Inherit: Same as first input
  Sum : Sum  Inputs=+-  SaturateOnIntegerOverflow=on  InputSameDT=on  OutDataTypeStr=Inherit: Same as first input
  Sum2 : Sum  Inputs=+-  SaturateOnIntegerOverflow=on  InputSameDT=on  OutDataTypeStr=Inherit: Same as first input
  aa : Outport
  wires:
  Demux/1 -> Product/1, Cubica/1(X1), Mux/1  "xySlope1"
  Demux/7 -> Product1/1, Cubica1/4(X2), Mux/3  "xySlope7"
  Demux/3 -> Product/2, Mux/4, Cubica/3(Slope1)  "xySlope3"
  Demux/2 -> Sum/1, Cubica/2(Y1)  "xySlope2"
  Demux/5 -> Cubica/5(Y2), Cubica1/2(Y1)  "xySlope5"
  Demux/6 -> Cubica/6(Slope2), Cubica1/3(Slope1)  "xySlope6"
  Demux/8 -> Sum2/1, Cubica1/5(Y2)  "xySlope8"
  Demux/9 -> Product1/2, Mux/14, Cubica1/6(Slope2)  "xySlope9"
  Demux/4 -> Cubica/4(X2), Cubica1/1(X1), Mux/2  "xySlope4"
  Product/1 -> Sum/2  ";"
  Sum/1 -> Mux/5  "aa)=xyslope(2)-xyslope(3)*xyslope(1)"
  Cubica/1(a1) -> Mux/6
  Cubica/2(a2) -> Mux/7
  Cubica/3(a3) -> Mux/8
  Cubica/4(a4) -> Mux/9
  Cubica1/1(a1) -> Mux/10
  Cubica1/2(a2) -> Mux/11
  Cubica1/3(a3) -> Mux/12
  Cubica1/4(a4) -> Mux/13
  Product1/1 -> Sum2/2
  Sum2/1 -> Mux/15  "aa15=xyslope8-xyslope9*xyslope7"
  X1/1 -> Demux/1
  Mux/1 -> aa/1

== system GuytonModel1986All_R2015a/Myogenic Autoregulation of Afferent Arteriole/function MyogenResp(PDIFF) - spline interpolation/Subsystem ==
  x : Inport
  aa : Inport  Port=2
  Demux : Demux  Outputs=15
  If : If  NumInputs=4  IfExpression=u1 <=u2  ElseIfExpressions=u1<=u3,u1<=u4
  If Action Subsystem : Subsystem  TreatAsAtomicUnit=on
  If Action Subsystem1 : Subsystem  TreatAsAtomicUnit=on
  If Action Subsystem2 : Subsystem  TreatAsAtomicUnit=on
  If Action Subsystem3 : Subsystem  TreatAsAtomicUnit=on
  Merge : Merge  Inputs=4
  y : Outport
  wires:
  x/1 -> If Action Subsystem3/1(x), If Action Subsystem2/1(x), If Action Subsystem1/1(x), If Action Subsystem/1(x), If/1
  Demux/1 -> If/2
  Merge/1 -> y/1
  If/1 -> If Action Subsystem/Action
  If/2 -> If Action Subsystem1/Action
  If/3 -> If Action Subsystem2/Action
  Demux/6 -> If Action Subsystem1/2(aa6)
  Demux/7 -> If Action Subsystem1/3(aa7)
  Demux/8 -> If Action Subsystem1/4(aa8)
  Demux/9 -> If Action Subsystem1/5(aa9)
  Demux/10 -> If Action Subsystem2/2(aa10)
  Demux/11 -> If Action Subsystem2/3(aa11)
  Demux/12 -> If Action Subsystem2/4(aa12)
  Demux/13 -> If Action Subsystem2/5(aa13)
  If/4 -> If Action Subsystem3/Action
  Demux/15 -> If Action Subsystem3/3(aa15)
  Demux/14 -> If Action Subsystem3/2(aa14)
  If Action Subsystem3/1(Out1) -> Merge/4
  If Action Subsystem2/1(y) -> Merge/3
  If Action Subsystem1/1(y) -> Merge/2
  If Action Subsystem/1(y) -> Merge/1
  Demux/2 -> If/3
  Demux/3 -> If/4
  Demux/4 -> If Action Subsystem/2(aa4)
  Demux/5 -> If Action Subsystem/3("aa6 ")
  aa/1 -> Demux/1

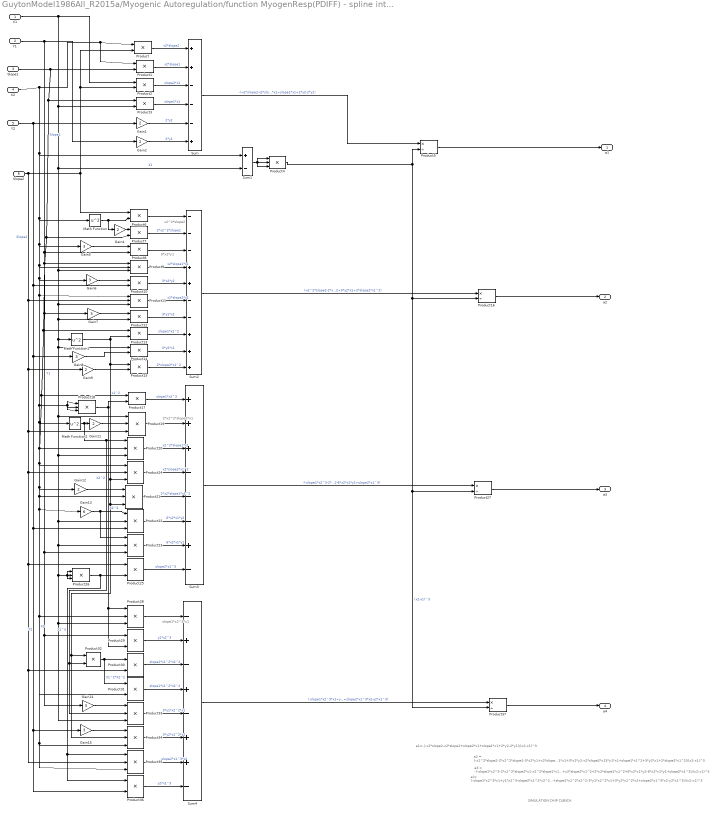
== system GuytonModel1986All_R2015a/Myogenic Autoregulation/function MyogenResp(PDIFF) - spline interpolation/If Action Subsystem/Cubica ==
  note: SIMULATION CHIP CUBICA
  note: a)= (-slope1*x2^3*x1+y1*x2^3-slope2*x1^2*x2^2+slope1*x1^2*x2^2-3*y1*x2^2*x1+3*y2*x1^2*x2+slope2*x1^3*x2-y2*x1^3)/(x2-x1)^3
  note: a3 = -(-slope1*x2^3-2*x2^2*slope2*x1-x2^2*slope1*x1+x2*slope2*x1^2+2*x2*slope1*x1^2+6*x2*x1*y2-6*x2*x1*y1+slope2*x1^3)/(x2-x1)^3
  note: a2 = (-x2^2*slope2-2*x2^2*slope1-3*x2*y1+x2*slope1*x1+3*x2*y2-x2*slope2*x13*y1*x1+slope1*x1^2+3*y2*x1+2*slope2*x1^2)/(x2-x1)^3
  note: slope1*x2^3*x1
  note: 2*x2^2*slope2*x1
  note: 3*x2*y1
  note: x2^2*slope2
  note: a1=-(-x2*slope2-x2*slope1+slope2*x1+slope1*x1+2*y2-2*y1)/(x2-x1)^3
  X1 : Inport
  Y1 : Inport  Port=2
  Slope1 : Inport  Port=3
  X2 : Inport  Port=4
  Y2 : Inport  Port=5
  Slope2 : Inport  Port=6
  Gain{1..2,4,9,11..12} (6 alike) : Gain  Gain=2  SaturateOnIntegerOverflow=on  OutDataTypeStr=Inherit: Same as input  ParamDataTypeStr=Inherit: Same as input
  Gain13 : Gain  Gain=6  SaturateOnIntegerOverflow=on  OutDataTypeStr=Inherit: Same as input  ParamDataTypeStr=Inherit: Same as input
  Gain{5..8,14..15} (6 alike) : Gain  Gain=3  SaturateOnIntegerOverflow=on  OutDataTypeStr=Inherit: Same as input  ParamDataTypeStr=Inherit: Same as input
  Math Function : Math  Operator=square  SaturateOnIntegerOverflow=on
  Math Function1 : Math  Operator=square  SaturateOnIntegerOverflow=on
  Math Function2 : Math  Operator=square  SaturateOnIntegerOverflow=on
  Product{,1..3,6..8,10,12..15,17,25,29..32,36} (19 alike) : Product  SaturateOnIntegerOverflow=on  InputSameDT=on  OutDataTypeStr=Inherit: Same as first input
  Product{4,9,11,18..24,26,28,33..35} (15 alike) : Product  Inputs=3  SaturateOnIntegerOverflow=on  InputSameDT=on  OutDataTypeStr=Inherit: Same as first input
  Product{5,16,27,37} (4 alike) : Product  Inputs=*/  SaturateOnIntegerOverflow=on  InputSameDT=on  OutDataTypeStr=Inherit: Same as first input
  Sum : Sum  Inputs=++---+  SaturateOnIntegerOverflow=on  InputSameDT=on  OutDataTypeStr=Inherit: Same as first input
  Sum1 : Sum  Inputs=+-  SaturateOnIntegerOverflow=on  InputSameDT=on  OutDataTypeStr=Inherit: Same as first input
  Sum2 : Sum  Inputs=---++--+++  SaturateOnIntegerOverflow=on  InputSameDT=on  OutDataTypeStr=Inherit: Same as first input
  Sum3 : Sum  Inputs=+++---+-  SaturateOnIntegerOverflow=on  InputSameDT=on  OutDataTypeStr=Inherit: Same as first input
  Sum4 : Sum  Inputs=-+-+-++-  SaturateOnIntegerOverflow=on  InputSameDT=on  OutDataTypeStr=Inherit: Same as first input
  a1 : Outport
  a2 : Outport  Port=2
  a3 : Outport  Port=3
  a4 : Outport  Port=4
  wires:
  Sum3/1 -> Product27/1  "-(-slope1*x2^3-2*x2^2*slope2*x1-x2^2*slope1*x1+x2*slope2*x1^2+2*x2*slope1*x1^2+6*x2*x1*y2-6*x2*x1*y1+slope2*x1^3)"
  Product37/1 -> a4/1
  Sum4/1 -> Product37/1  "(-slope1*x2^3*x1+y1*x2^3-slope2*x1^2*x2^2+slope1*x1^2*x2^2-3*y1*x2^2*x1+3*y2*x1^2*x2+slope2*x1^3*x2-y2*x1^3)"
  Product36/1 -> Sum4/8  "y2*x1^3"
  Product35/1 -> Sum4/7  "slope2*x1^3*x2"
  Gain15/1 -> Product34/1
  Product34/1 -> Sum4/6  "3*y2*x1^2*x2"
  Gain14/1 -> Product33/1
  Product33/1 -> Sum4/5  "3*y1*x2^2*x1"
  Product32/1 -> Product31/1, Product30/1  "X1^2*X2^2"
  Product31/1 -> Sum4/4  "slope1*x1^2*x2^2"
  Product30/1 -> Sum4/3  "slope2*x1^2*x2^2"
  Product29/1 -> Sum4/2  "y1*x2^3"
  Product28/1 -> Sum4/1
  Product27/1 -> a3/1
  Product26/1 -> Product36/1, Product35/1, Product25/2  "X1^3"
  Product25/1 -> Sum3/8  "slope2*x1^3"
  Product24/1 -> Sum3/4  "x2*slope2*x1^2"
  Product21/1 -> Sum3/5  "2*x2*slope1*x1^2"
  Product22/1 -> Sum3/6  "6*x2*x1*y2"
  Product23/1 -> Sum3/7  "6*x2*x1*y1"
  Gain13/1 -> Product23/1, Product22/1
  Gain12/1 -> Product21/1
  Product20/1 -> Sum3/3  "x2^2*slope1*x1"
  Gain11/1 -> Product19/2
  Math Function2/1 -> Product33/2, Product32/2, Product20/1, Gain11/1  "X2^2"
  Product19/1 -> Sum3/2
  Product18/1 -> Product29/2, Product28/1, Product17/2  "X2^3"
  Product17/1 -> Sum3/1  "slope1*x2^3"
  Product16/1 -> a2/1
  Sum2/1 -> Product16/1  "(-x2^2*slope2-2*x2^2*slope1-3*x2*y1+x2*slope1*x1+3*x2*y2-x2*slope2*x1-3*y1*x1+slope1*x1^2+3*y2*x1+2*slope2*x1^2)"
  Gain9/1 -> Product15/2
  Product15/1 -> Sum2/10  "2*slope2*x1^2"
  Gain8/1 -> Product14/2
  Product14/1 -> Sum2/9  "3*y2*x1"
  Math Function1/1 -> Product34/2, Product32/1, Product21/3, Product24/3, Product15/1, Product13/2  "x1^2"
  Product13/1 -> Sum2/8  "slope1*x1^2"
  Gain7/1 -> Product12/1
  Product12/1 -> Sum2/7  "3*y1*x1"
  Product11/1 -> Sum2/6  "x2*slope2*x1"
  Product10/1 -> Sum2/5  "3*x2*y2"
  Gain6/1 -> Product10/1
  Product9/1 -> Sum2/4  "x2*slope1*x1"
  Gain5/1 -> Product8/1
  Product8/1 -> Sum2/3
  Product7/1 -> Sum2/2  "2*x2^2*slope1"
  Gain4/1 -> Product7/1
  Product6/1 -> Sum2/1
  Math Function/1 -> Gain4/1, Product6/2
  Product5/1 -> a1/1
  Product4/1 -> Product37/2, Product27/2, Product16/2, Product5/2  "(x2-x1)^3"
  Sum1/1 -> Product4/1, Product4/3, Product4/2
  Sum/1 -> Product5/1  "-(-x2*slope2-x2*slope1+slope2*x1+slope1*x1+2*y2-2*y1)"
  Y1/1 -> Gain14/1, Product29/1, Product23/3, Gain7/1, Product8/2, Gain2/1  "Y1"
  Gain2/1 -> Sum/6  "2*y1"
  Gain1/1 -> Sum/5  "2*y2"
  Y2/1 -> Product36/2, Gain15/1, Product22/3, Gain8/1, Product10/2, Gain1/1  "Y2"
  Product3/1 -> Sum/4  "slope1*x1"
  Product2/1 -> Sum/3  "slope2*x1"
  X1/1 -> Sum1/2, Product33/3, Product28/3, Product26/1, Product26/3, Product26/2, Product23/2, Product22/2, Product20/3, Product19/1, Product14/1, Math Function1/1, Product12/2, Product11/3, Product9/3, Product3/2, Product2/1  "X1"
  Product1/1 -> Sum/2  "x2*slope1"
  Product/1 -> Sum/1  "x2*slope2"
  Slope1/1 -> Product31/2, Product28/2, Product21/2, Product20/2, Product17/1, Product13/1, Product9/1, Product7/2, Product3/1, Product1/2  "Slope1"
  Slope2/1 -> Product35/2, Product30/2, Product25/1, Product24/2, Product19/3, Gain9/1, Product11/2, Product6/1, Product2/2, Product/2  "Slope2"
  X2/1 -> Product/1, Product1/1, Product24/1, Product35/3, Product34/3, Gain13/1, Gain12/1, Math Function2/1, Product18/3, Product18/1, Product18/2, Product11/1, Gain6/1, Product9/2, Gain5/1, Math Function/1, Sum1/1  "X2"

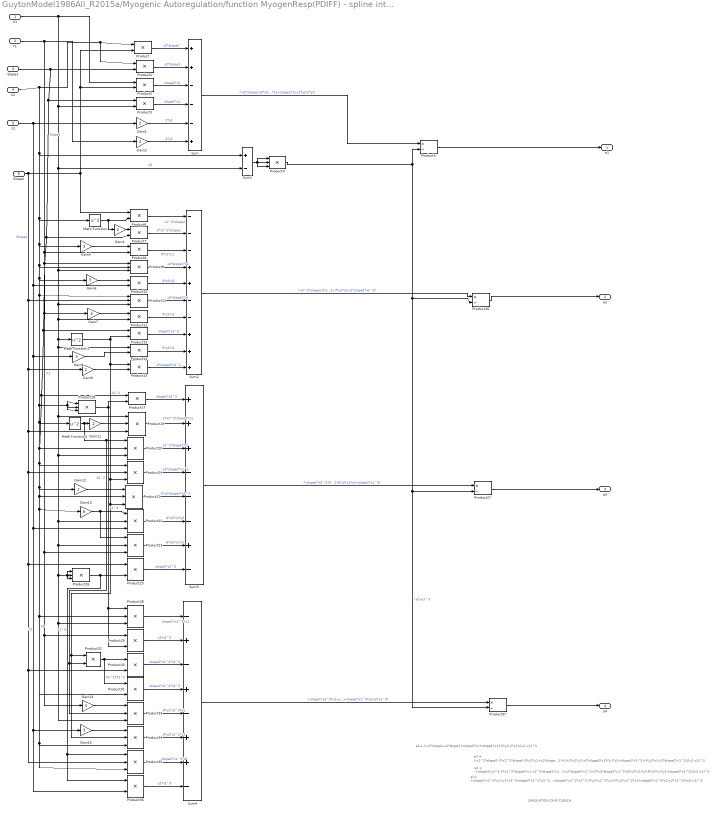
== system GuytonModel1986All_R2015a/Myogenic Autoregulation/function MyogenResp(PDIFF) - spline interpolation/If Action Subsystem/Cubica1 ==
  note: SIMULATION CHIP CUBICA
  note: a)= (-slope1*x2^3*x1+y1*x2^3-slope2*x1^2*x2^2+slope1*x1^2*x2^2-3*y1*x2^2*x1+3*y2*x1^2*x2+slope2*x1^3*x2-y2*x1^3)/(x2-x1)^3
  note: a3 = -(-slope1*x2^3-2*x2^2*slope2*x1-x2^2*slope1*x1+x2*slope2*x1^2+2*x2*slope1*x1^2+6*x2*x1*y2-6*x2*x1*y1+slope2*x1^3)/(x2-x1)^3
  note: a2 = (-x2^2*slope2-2*x2^2*slope1-3*x2*y1+x2*slope1*x1+3*x2*y2-x2*slope2*x13*y1*x1+slope1*x1^2+3*y2*x1+2*slope2*x1^2)/(x2-x1)^3
  note: slope1*x2^3*x1
  note: 2*x2^2*slope2*x1
  note: 3*x2*y1
  note: x2^2*slope2
  note: a1=-(-x2*slope2-x2*slope1+slope2*x1+slope1*x1+2*y2-2*y1)/(x2-x1)^3
  X1 : Inport
  Y1 : Inport  Port=2
  Slope1 : Inport  Port=3
  X2 : Inport  Port=4
  Y2 : Inport  Port=5
  Slope2 : Inport  Port=6
  Gain{1..2,4,9,11..12} (6 alike) : Gain  Gain=2  SaturateOnIntegerOverflow=on  OutDataTypeStr=Inherit: Same as input  ParamDataTypeStr=Inherit: Same as input
  Gain13 : Gain  Gain=6  SaturateOnIntegerOverflow=on  OutDataTypeStr=Inherit: Same as input  ParamDataTypeStr=Inherit: Same as input
  Gain{5..8,14..15} (6 alike) : Gain  Gain=3  SaturateOnIntegerOverflow=on  OutDataTypeStr=Inherit: Same as input  ParamDataTypeStr=Inherit: Same as input
  Math Function : Math  Operator=square  SaturateOnIntegerOverflow=on
  Math Function1 : Math  Operator=square  SaturateOnIntegerOverflow=on
  Math Function2 : Math  Operator=square  SaturateOnIntegerOverflow=on
  Product{,1..3,6..8,10,12..15,17,25,29..32,36} (19 alike) : Product  SaturateOnIntegerOverflow=on  InputSameDT=on  OutDataTypeStr=Inherit: Same as first input
  Product{4,9,11,18..24,26,28,33..35} (15 alike) : Product  Inputs=3  SaturateOnIntegerOverflow=on  InputSameDT=on  OutDataTypeStr=Inherit: Same as first input
  Product{5,16,27,37} (4 alike) : Product  Inputs=*/  SaturateOnIntegerOverflow=on  InputSameDT=on  OutDataTypeStr=Inherit: Same as first input
  Sum : Sum  Inputs=++---+  SaturateOnIntegerOverflow=on  InputSameDT=on  OutDataTypeStr=Inherit: Same as first input
  Sum1 : Sum  Inputs=+-  SaturateOnIntegerOverflow=on  InputSameDT=on  OutDataTypeStr=Inherit: Same as first input
  Sum2 : Sum  Inputs=---++--+++  SaturateOnIntegerOverflow=on  InputSameDT=on  OutDataTypeStr=Inherit: Same as first input
  Sum3 : Sum  Inputs=+++---+-  SaturateOnIntegerOverflow=on  InputSameDT=on  OutDataTypeStr=Inherit: Same as first input
  Sum4 : Sum  Inputs=-+-+-++-  SaturateOnIntegerOverflow=on  InputSameDT=on  OutDataTypeStr=Inherit: Same as first input
  a1 : Outport
  a2 : Outport  Port=2
  a3 : Outport  Port=3
  a4 : Outport  Port=4
  wires:
  Sum3/1 -> Product27/1  "-(-slope1*x2^3-2*x2^2*slope2*x1-x2^2*slope1*x1+x2*slope2*x1^2+2*x2*slope1*x1^2+6*x2*x1*y2-6*x2*x1*y1+slope2*x1^3)"
  Product37/1 -> a4/1
  Sum4/1 -> Product37/1  "(-slope1*x2^3*x1+y1*x2^3-slope2*x1^2*x2^2+slope1*x1^2*x2^2-3*y1*x2^2*x1+3*y2*x1^2*x2+slope2*x1^3*x2-y2*x1^3)"
  Product36/1 -> Sum4/8  "y2*x1^3"
  Product35/1 -> Sum4/7  "slope2*x1^3*x2"
  Gain15/1 -> Product34/1
  Product34/1 -> Sum4/6  "3*y2*x1^2*x2"
  Gain14/1 -> Product33/1
  Product33/1 -> Sum4/5  "3*y1*x2^2*x1"
  Product32/1 -> Product31/1, Product30/1  "X1^2*X2^2"
  Product31/1 -> Sum4/4  "slope1*x1^2*x2^2"
  Product30/1 -> Sum4/3  "slope2*x1^2*x2^2"
  Product29/1 -> Sum4/2  "y1*x2^3"
  Product28/1 -> Sum4/1
  Product27/1 -> a3/1
  Product26/1 -> Product36/1, Product35/1, Product25/2  "X1^3"
  Product25/1 -> Sum3/8  "slope2*x1^3"
  Product24/1 -> Sum3/4  "x2*slope2*x1^2"
  Product21/1 -> Sum3/5  "2*x2*slope1*x1^2"
  Product22/1 -> Sum3/6  "6*x2*x1*y2"
  Product23/1 -> Sum3/7  "6*x2*x1*y1"
  Gain13/1 -> Product23/1, Product22/1
  Gain12/1 -> Product21/1
  Product20/1 -> Sum3/3  "x2^2*slope1*x1"
  Gain11/1 -> Product19/2
  Math Function2/1 -> Product33/2, Product32/2, Product20/1, Gain11/1  "X2^2"
  Product19/1 -> Sum3/2
  Product18/1 -> Product29/2, Product28/1, Product17/2  "X2^3"
  Product17/1 -> Sum3/1  "slope1*x2^3"
  Product16/1 -> a2/1
  Sum2/1 -> Product16/1  "(-x2^2*slope2-2*x2^2*slope1-3*x2*y1+x2*slope1*x1+3*x2*y2-x2*slope2*x1-3*y1*x1+slope1*x1^2+3*y2*x1+2*slope2*x1^2)"
  Gain9/1 -> Product15/2
  Product15/1 -> Sum2/10  "2*slope2*x1^2"
  Gain8/1 -> Product14/2
  Product14/1 -> Sum2/9  "3*y2*x1"
  Math Function1/1 -> Product34/2, Product32/1, Product21/3, Product24/3, Product15/1, Product13/2  "x1^2"
  Product13/1 -> Sum2/8  "slope1*x1^2"
  Gain7/1 -> Product12/1
  Product12/1 -> Sum2/7  "3*y1*x1"
  Product11/1 -> Sum2/6  "x2*slope2*x1"
  Product10/1 -> Sum2/5  "3*x2*y2"
  Gain6/1 -> Product10/1
  Product9/1 -> Sum2/4  "x2*slope1*x1"
  Gain5/1 -> Product8/1
  Product8/1 -> Sum2/3
  Product7/1 -> Sum2/2  "2*x2^2*slope1"
  Gain4/1 -> Product7/1
  Product6/1 -> Sum2/1
  Math Function/1 -> Gain4/1, Product6/2
  Product5/1 -> a1/1
  Product4/1 -> Product37/2, Product27/2, Product16/2, Product5/2  "(x2-x1)^3"
  Sum1/1 -> Product4/1, Product4/3, Product4/2
  Sum/1 -> Product5/1  "-(-x2*slope2-x2*slope1+slope2*x1+slope1*x1+2*y2-2*y1)"
  Y1/1 -> Gain14/1, Product29/1, Product23/3, Gain7/1, Product8/2, Gain2/1  "Y1"
  Gain2/1 -> Sum/6  "2*y1"
  Gain1/1 -> Sum/5  "2*y2"
  Y2/1 -> Product36/2, Gain15/1, Product22/3, Gain8/1, Product10/2, Gain1/1  "Y2"
  Product3/1 -> Sum/4  "slope1*x1"
  Product2/1 -> Sum/3  "slope2*x1"
  X1/1 -> Sum1/2, Product33/3, Product28/3, Product26/1, Product26/3, Product26/2, Product23/2, Product22/2, Product20/3, Product19/1, Product14/1, Math Function1/1, Product12/2, Product11/3, Product9/3, Product3/2, Product2/1  "X1"
  Product1/1 -> Sum/2  "x2*slope1"
  Product/1 -> Sum/1  "x2*slope2"
  Slope1/1 -> Product31/2, Product28/2, Product21/2, Product20/2, Product17/1, Product13/1, Product9/1, Product7/2, Product3/1, Product1/2  "Slope1"
  Slope2/1 -> Product35/2, Product30/2, Product25/1, Product24/2, Product19/3, Gain9/1, Product11/2, Product6/1, Product2/2, Product/2  "Slope2"
  X2/1 -> Product/1, Product1/1, Product24/1, Product35/3, Product34/3, Gain13/1, Gain12/1, Math Function2/1, Product18/3, Product18/1, Product18/2, Product11/1, Gain6/1, Product9/2, Gain5/1, Math Function/1, Sum1/1  "X2"

== system GuytonModel1986All_R2015a/Myogenic Autoregulation/function MyogenResp(PDIFF) - spline interpolation/Subsystem/If Action Subsystem ==
  x : Inport
  aa4 : Inport  Port=2
  "aa6 " : Inport  Port=3
  Action Port : ActionPort  ActionType=then
  Product : Product  SaturateOnIntegerOverflow=on  InputSameDT=on  OutDataTypeStr=Inherit: Same as first input
  Sum : Sum  SaturateOnIntegerOverflow=on  InputSameDT=on  OutDataTypeStr=Inherit: Same as first input
  y : Outport
  wires:
  Sum/1 -> y/1  "y=aa4*x+aa5"
  "aa6 "/1 -> Sum/2
  Product/1 -> Sum/1
  x/1 -> Product/1
  aa4/1 -> Product/2

== system GuytonModel1986All_R2015a/Myogenic Autoregulation/function MyogenResp(PDIFF) - spline interpolation/Subsystem/If Action Subsystem1 ==
  x : Inport
  aa6 : Inport  Port=2
  aa7 : Inport  Port=3
  aa8 : Inport  Port=4
  aa9 : Inport  Port=5
  Action Port : ActionPort  ActionType=elseif
  Math Function : Math  Operator=square  SaturateOnIntegerOverflow=on
  Product : Product  Inputs=3  SaturateOnIntegerOverflow=on  InputSameDT=on  OutDataTypeStr=Inherit: Same as first input
  Product2 : Product  SaturateOnIntegerOverflow=on  InputSameDT=on  OutDataTypeStr=Inherit: Same as first input
  Product3 : Product  SaturateOnIntegerOverflow=on  InputSameDT=on  OutDataTypeStr=Inherit: Same as first input
  Sum : Sum  Inputs=++++  SaturateOnIntegerOverflow=on  InputSameDT=on  OutDataTypeStr=Inherit: Same as first input
  y : Outport
  wires:
  Sum/1 -> y/1  "y=aa6*x^3+aa7*x^2+aa8*x+aa9"
  aa9/1 -> Sum/4
  Product3/1 -> Sum/3
  aa8/1 -> Product3/2
  Product2/1 -> Sum/2
  aa7/1 -> Product2/2
  aa6/1 -> Product/3
  Product/1 -> Sum/1
  Math Function/1 -> Product2/1, Product/1
  x/1 -> Product3/1, Product/2, Math Function/1

== system GuytonModel1986All_R2015a/Myogenic Autoregulation/function MyogenResp(PDIFF) - spline interpolation/Subsystem/If Action Subsystem2 ==
  x : Inport
  aa10 : Inport  Port=2
  aa11 : Inport  Port=3
  aa12 : Inport  Port=4
  aa13 : Inport  Port=5
  Action Port : ActionPort  ActionType=elseif
  Math Function : Math  Operator=square  SaturateOnIntegerOverflow=on
  Product : Product  Inputs=3  SaturateOnIntegerOverflow=on  InputSameDT=on  OutDataTypeStr=Inherit: Same as first input
  Product2 : Product  SaturateOnIntegerOverflow=on  InputSameDT=on  OutDataTypeStr=Inherit: Same as first input
  Product3 : Product  SaturateOnIntegerOverflow=on  InputSameDT=on  OutDataTypeStr=Inherit: Same as first input
  Sum : Sum  Inputs=++++  SaturateOnIntegerOverflow=on  InputSameDT=on  OutDataTypeStr=Inherit: Same as first input
  y : Outport
  wires:
  x/1 -> Math Function/1, Product/2, Product3/1
  Math Function/1 -> Product/1, Product2/1
  Product/1 -> Sum/1
  aa10/1 -> Product/3
  aa11/1 -> Product2/2
  Product2/1 -> Sum/2
  aa12/1 -> Product3/2
  Product3/1 -> Sum/3
  aa13/1 -> Sum/4
  Sum/1 -> y/1  "y=aa6*x^3+aa7*x^2+aa8*x+aa9"

== system GuytonModel1986All_R2015a/Myogenic Autoregulation/function MyogenResp(PDIFF) - spline interpolation/Subsystem/If Action Subsystem3 ==
  x : Inport
  aa14 : Inport  Port=2
  aa15 : Inport  Port=3
  Action Port : ActionPort  ActionType=else
  Product3 : Product  SaturateOnIntegerOverflow=on  InputSameDT=on  OutDataTypeStr=Inherit: Same as first input
  Sum : Sum  SaturateOnIntegerOverflow=on  InputSameDT=on  OutDataTypeStr=Inherit: Same as first input
  Out1 : Outport
  wires:
  Sum/1 -> Out1/1
  Product3/1 -> Sum/1
  aa15/1 -> Sum/2
  x/1 -> Product3/1
  aa14/1 -> Product3/2
